simulink model "discrete"  (R2018b)
settings: Solver=VariableStepAuto  StartTime=0.0  StopTime=10.0  RelTol=1e-3
settings Model: Creator=aycfink  LastModifiedBy=aycfink

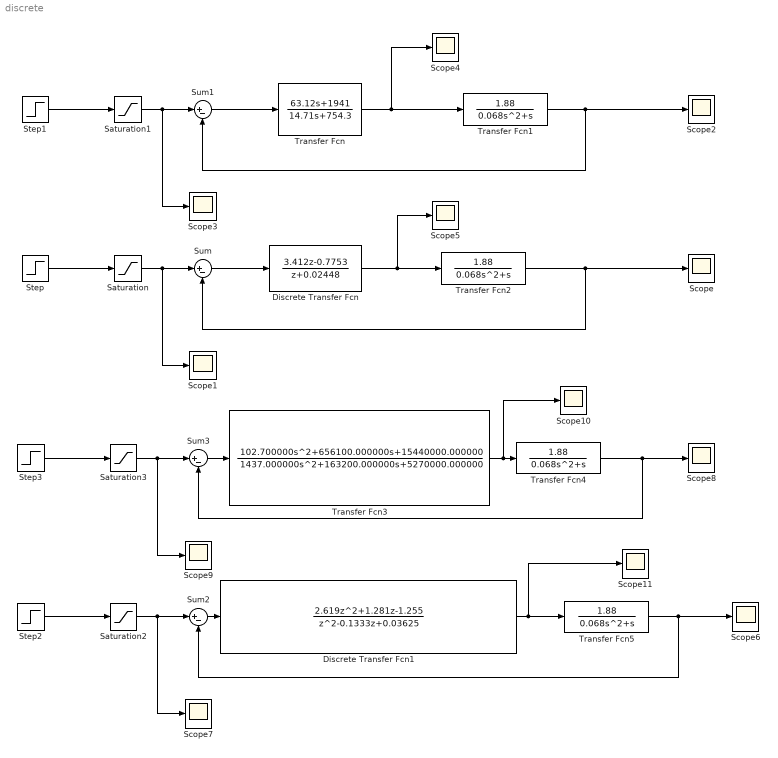
== system discrete ==
  Discrete Transfer Fcn : DiscreteTransferFcn  Numerator=[3.412 -0.7753]  Denominator=[1 0.02448]  SampleTime=0.040948
  Discrete Transfer Fcn1 : DiscreteTransferFcn  Numerator=[2.619 1.281 -1.255]  Denominator=[1 -0.1333 0.03625]  SampleTime=0.029012
  Saturation{,1..3} (4 alike) : Saturate  UpperLimit=0.7  LowerLimit=-0.7
  Scope{,1..11} (12 alike) : Scope
  Step{,1..3} (4 alike) : Step  Time=5  Before=-0.7  After=0.7  SampleTime=0
  Sum{,1..3} (4 alike) : Sum  Inputs=|+-
  Transfer Fcn : TransferFcn  Numerator=[63.12 1941]  Denominator=[14.71 754.3]
  Transfer Fcn{1..2,4..5} (4 alike) : TransferFcn  Numerator=[1.88]  Denominator=[0.068 1 0]
  Transfer Fcn3 : TransferFcn  Numerator=[102.700000 656100.000000 15440000.000000]  Denominator=[1437.000000 163200.000000 5270000.000000]
  wires:
  Discrete Transfer Fcn/1 -> Transfer Fcn2/1, Scope5/1
  Transfer Fcn2/1 -> Sum/2, Scope/1
  Sum/1 -> Discrete Transfer Fcn/1
  Saturation/1 -> Scope1/1, Sum/1
  Step/1 -> Saturation/1
  Transfer Fcn1/1 -> Sum1/2, Scope2/1
  Transfer Fcn/1 -> Transfer Fcn1/1, Scope4/1
  Saturation1/1 -> Scope3/1, Sum1/1
  Sum1/1 -> Transfer Fcn/1
  Step1/1 -> Saturation1/1
  Saturation2/1 -> Scope7/1, Sum2/1
  Step3/1 -> Saturation3/1
  Saturation3/1 -> Scope9/1, Sum3/1
  Transfer Fcn4/1 -> Sum3/2, Scope8/1
  Transfer Fcn5/1 -> Sum2/2, Scope6/1
  Transfer Fcn3/1 -> Scope10/1, Transfer Fcn4/1
  Sum3/1 -> Transfer Fcn3/1
  Discrete Transfer Fcn1/1 -> Scope11/1, Transfer Fcn5/1
  Sum2/1 -> Discrete Transfer Fcn1/1
  Step2/1 -> Saturation2/1
